simulink model "Collision_avoidance"  (R2020a)
settings: Solver=FixedStepAuto  StartTime=0.0  StopTime=180  FixedStep=0.01  RelTol=1e-3
libraries: simulink x2
settings Model: Creator=Santo  LastModifiedBy=apoor
settings DataIOCC: ReturnWorkspaceOutputs=off
settings OptimizationCC: LifeSpan=inf
settings DebuggingCC: ArithmeticOperatorsInVariantConditions=warning
settings HardwareCC: ProdBitPerSizeT=32  ProdBitPerPtrDiffT=32  ProdWordSize=32  ProdHWDeviceType=Specified
settings SFSimCC: SimUseLocalCustomCode=off  CustomCodeUndefinedFunction=UseInterfaceOnly
settings RTWCC: RTWUseLocalCustomCode=off
settings CodeAppCC: StateflowObjectComments=on

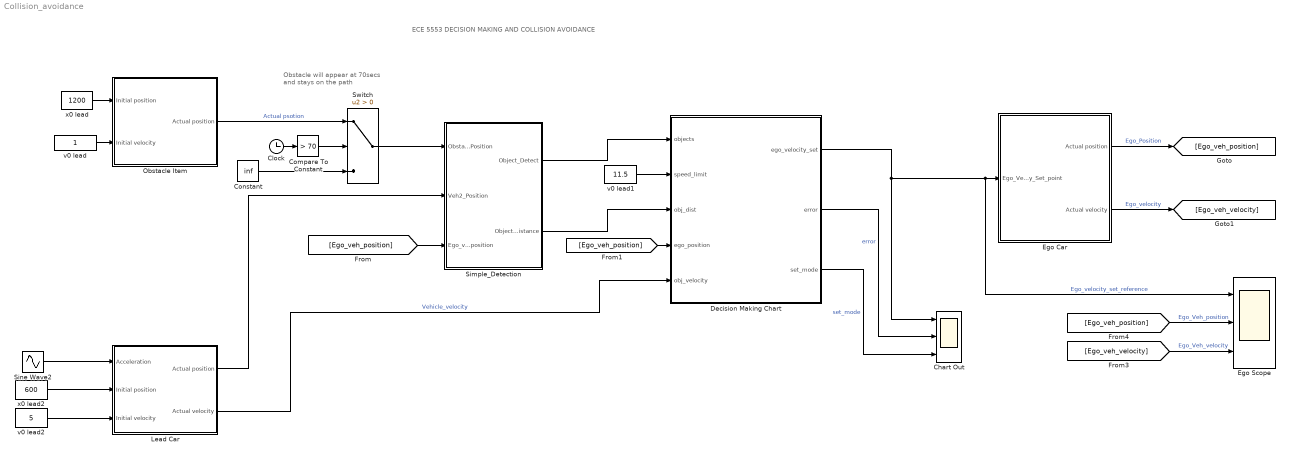
== system Collision_avoidance ==
  note: ECE 5553 DECISION MAKING AND COLLISION AVOIDANCE
  note: Obstacle will appear at 70secs and stays on the path
  Chart Out : Scope  NumInputPorts=3
  Clock : Clock
  Compare To Constant : simulink/Logic and Bit Operations/Compare To Constant  relop=>  const=70  OutDataTypeStr=boolean
  Constant : Constant  Value=inf
  Decision Making Chart : Stateflow chart  TreatAsAtomicUnit=on
  Ego Car : Subsystem
  Ego Scope : Scope  NumInputPorts=3
  Lead Car : Subsystem
  Obstacle Item : Subsystem
  Simple_Detection : Subsystem
  Sine Wave2 : Sin  Amplitude=5  Frequency=0.5  SampleTime=0
  Switch : Switch  Criteria=u2 > Threshold
  v0 lead : Constant  SampleTime=0
  v0 lead1 : Constant  Value=11.5  SampleTime=0
  v0 lead2 : Constant  Value=5  SampleTime=0
  x0 lead : Constant  Value=1200  SampleTime=0
  x0 lead2 : Constant  Value=600  SampleTime=0
  wires:
  x0 lead/1 -> Obstacle Item/1(Initial position)
  v0 lead/1 -> Obstacle Item/2(Initial velocity)
  Lead Car/1(Actual position) -> Simple_Detection/2(Veh2_Position)
  x0 lead2/1 -> Lead Car/2(Initial position)
  v0 lead2/1 -> Lead Car/3(Initial velocity)
  Sine Wave2/1 -> Lead Car/1(Acceleration)
  Simple_Detection/1(Object_Detect) -> Decision Making Chart/1(objects)
  v0 lead1/1 -> Decision Making Chart/2(speed_limit)
  Decision Making Chart/1(ego_velocity_set) -> Chart Out/1, Ego Scope/1, Ego Car/1(Ego_Velocity_Set_point)  "Ego_velocity_set_reference"
  Ego Car/1(Actual position) -> [Ego_veh_position]  "Ego_Position"
  Ego Car/2(Actual velocity) -> [Ego_veh_velocity]  "Ego_velocity"
  Simple_Detection/2(Object_Relative_Distance) -> Decision Making Chart/3(obj_dist)
  Decision Making Chart/2(error) -> Chart Out/2  "error"
  [Ego_veh_position] -> Simple_Detection/3(Ego_veh_position)
  [Ego_veh_position] -> Decision Making Chart/4(ego_position)
  [Ego_veh_velocity] -> Ego Scope/3  "Ego_Veh_velocity"
  [Ego_veh_position] -> Ego Scope/2  "Ego_Veh_position"
  Decision Making Chart/3(set_mode) -> Chart Out/3  "set_mode"
  Lead Car/2(Actual velocity) -> Decision Making Chart/5(obj_velocity)  "Vehicle_velocity"
  Compare To Constant/1 -> Switch/2
  Switch/1 -> Simple_Detection/1(Obstacle_Position)
  Obstacle Item/1(Actual position) -> Switch/1  "Actual psotion"
  Constant/1 -> Switch/3
  Clock/1 -> Compare To Constant/1

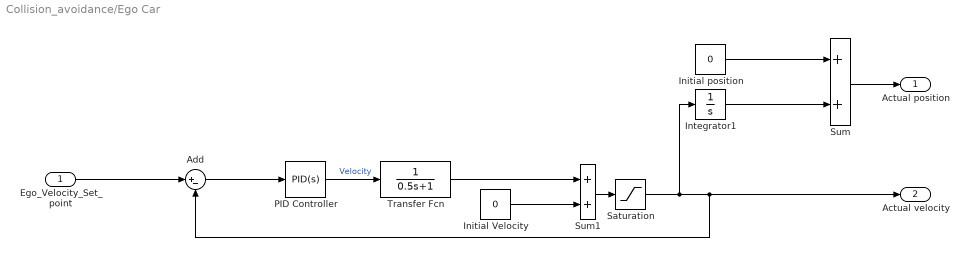
== system Collision_avoidance/Ego Car ==
  Ego_Velocity_Set_point : Inport
  Add : Sum  Inputs=|+-
  Initial Velocity : Constant  Value=0
  Initial position : Constant  Value=0
  Integrator1 : Integrator
  PID Controller : simulink/Continuous/PID Controller  Controller=PID  Form=Parallel  TimeDomain=Continuous-time  UseExternalTs=off  SampleTime=-1  IntegratorMethod=Forward Euler  FilterMethod=Forward Euler  ControllerParametersSource=internal  P=0.543871188851985  I=1.5579001255467  D=0  UseFilter=on  N=100  TunerSelectOption=Transfer Function Based (PID Tuner App)  InitialConditionSource=internal  InitialConditionForIntegrator=0  InitialConditionForFilter=0  DifferentiatorICPrevScaledInput=0  ExternalReset=none  TrackingMode=off  Kt=1  LimitOutput=off  UpperSaturationLimit=inf  LowerSaturationLimit=-inf  LinearizeAsGain=on  AntiWindupMode=none  Kb=1  POutMin=[]  POutMax=[]  IOutMin=[]  IOutMax=[]  DOutMin=[]  DOutMax=[]  NOutMin=[]  NOutMax=[]  SumOutMin=[]  SumOutMax=[]  SaturationOutMin=[]  SaturationOutMax=[]  PParamMin=[]  PParamMax=[]  IParamMin=[]  IParamMax=[]  DParamMin=[]  DParamMax=[]  NParamMin=[]  NParamMax=[]  KbParamMin=[]  KbParamMax=[]  KtParamMin=[]  KtParamMax=[]  KbOutMin=[]  KbOutMax=[]  KtOutMin=[]  KtOutMax=[]  IntegratorOutMin=[]  IntegratorOutMax=[]  FilterOutMin=[]  FilterOutMax=[]  SumI1OutMin=[]  SumI1OutMax=[]  SumI2OutMin=[]  SumI2OutMax=[]  SumI3OutMin=[]  SumI3OutMax=[]  SumI4OutMin=[]  SumI4OutMax=[]  SumDOutMin=[]  SumDOutMax=[]  DifferentiatorOutMin=[]  DifferentiatorOutMax=[]  FilterDiffOutCoefMin=[]  FilterDiffOutCoefMax=[]  ReciprocalOutMin=[]  ReciprocalOutMax=[]  SumDenOutMin=[]  SumDenOutMax=[]  SumNumOutMin=[]  SumNumOutMax=[]  DivideOutMin=[]  DivideOutMax=[]  UdiffTsProdOutMin=[]  UdiffTsProdOutMax=[]  NTsProdOutMin=[]  NTsProdOutMax=[]  UintegralTsProdOutMin=[]  UintegralTsProdOutMax=[]  UngainTsProdOutMin=[]  UngainTsProdOutMax=[]  IntegratorContinuousStateAttributes=''  IntegratorStateMustResolveToSignalObject=off  IntegratorRTWStateStorageClass=Auto  FilterContinuousStateAttributes=''  FilterStateMustResolveToSignalObject=off  FilterRTWStateStorageClass=Auto  ParallelPVariant=InternalParameters  IdealPVariant=Disabled  IVariant=InternalParameters  DVariant=InternalParameters  IntegratorVariant=Continuous  SatVariant=Disabled  AWVariant=Passthrough  PCopyVariant=Disabled  TRVariant=Disabled  FdbkBlocksVariant=Forward  IdealPFdbkVariant=Disabled  SatFdbkVariant=Disabled  DerivativeFilterVariant=ContFilter  NVariant=InternalParameters  NCopyVariant=Disabled  FilterICVariant=InternalICsFilter  IntegratorICVariant=InternalICs  ExternalResetVariant=Disabled  TRSumVariant=Passthrough  SumFdbkVariant=Disabled  SumVariant=Sum_PID  TsampFilterVariant=InternalTs  TsampNgainVariant=Passthrough  TsampIntegralVariant=Passthrough
  Saturation : Saturate  UpperLimit=inf  LowerLimit=0
  Sum : Sum
  Sum1 : Sum
  Transfer Fcn : TransferFcn  Denominator=[0.5 1]
  Actual position : Outport
  Actual velocity : Outport  Port=2
  wires:
  Transfer Fcn/1 -> Sum1/1
  Initial Velocity/1 -> Sum1/2
  Sum/1 -> Actual position/1
  Sum1/1 -> Saturation/1
  PID Controller/1 -> Transfer Fcn/1  "Velocity"
  Initial position/1 -> Sum/1
  Integrator1/1 -> Sum/2
  Add/1 -> PID Controller/1
  Ego_Velocity_Set_point/1 -> Add/1
  Saturation/1 -> Integrator1/1, Add/2, Actual velocity/1

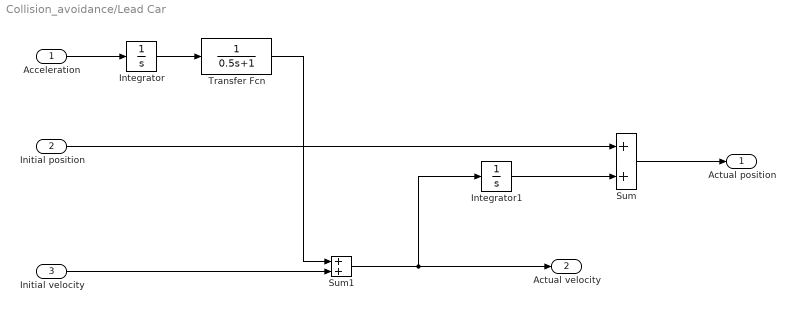
== system Collision_avoidance/Lead Car ==
  Acceleration : Inport
  Initial position : Inport  Port=2
  Initial velocity : Inport  Port=3
  Integrator : Integrator
  Integrator1 : Integrator
  Sum : Sum
  Sum1 : Sum
  Transfer Fcn : TransferFcn  Denominator=[0.5 1]
  Actual position : Outport
  Actual velocity : Outport  Port=2
  wires:
  Integrator1/1 -> Sum/2
  Initial position/1 -> Sum/1
  Acceleration/1 -> Integrator/1
  Sum1/1 -> Actual velocity/1, Integrator1/1
  Integrator/1 -> Transfer Fcn/1
  Sum/1 -> Actual position/1
  Initial velocity/1 -> Sum1/2
  Transfer Fcn/1 -> Sum1/1

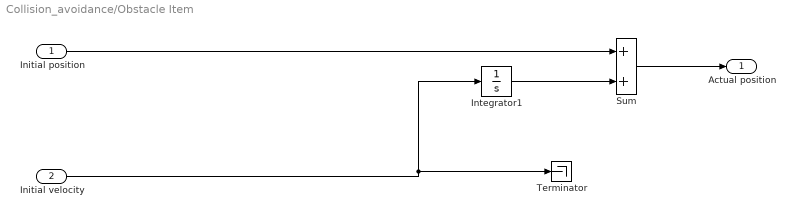
== system Collision_avoidance/Obstacle Item ==
  Initial position : Inport
  Initial velocity : Inport  Port=2
  Integrator1 : Integrator
  Sum : Sum
  Terminator : Terminator
  Actual position : Outport
  wires:
  Sum/1 -> Actual position/1
  Initial velocity/1 -> Terminator/1, Integrator1/1
  Initial position/1 -> Sum/1
  Integrator1/1 -> Sum/2

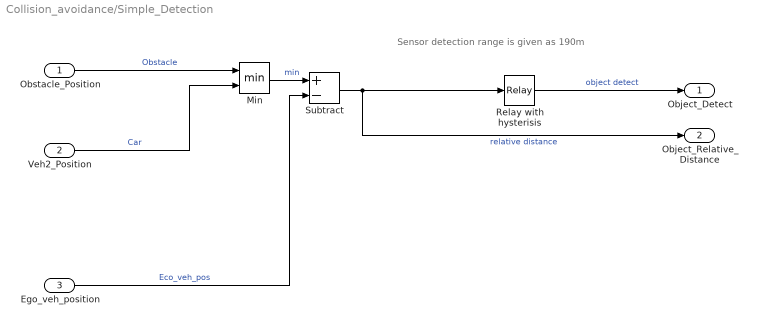
== system Collision_avoidance/Simple_Detection ==
  note: Sensor detection range is given as 190m
  Obstacle_Position : Inport
  Veh2_Position : Inport  Port=2
  Ego_veh_position : Inport  Port=3
  Min : MinMax  Inputs=2
  Relay with hysterisis : Relay  OnSwitchValue=210  OffSwitchValue=190  OnOutputValue=0  OffOutputValue=1
  Subtract : Sum  Inputs=+-
  Object_Detect : Outport
  Object_Relative_Distance : Outport  Port=2
  wires:
  Obstacle_Position/1 -> Min/1  "Obstacle"
  Veh2_Position/1 -> Min/2  "Car"
  Min/1 -> Subtract/1  "min"
  Ego_veh_position/1 -> Subtract/2  "Eco_veh_pos"
  Subtract/1 -> Relay with hysterisis/1, Object_Relative_Distance/1  "relative distance"
  Relay with hysterisis/1 -> Object_Detect/1  "object detect"

== stateflow chart Collision_avoidance/Decision Making Chart ==
  state Follow_Speed_Limit
    ego_velocity_set=speed_limit;
    set_mode=0;
  state objects
  state Lead_Velocity1
    ego_velocity_set=obj_velocity;
    set_mode=1
  state Relative_Distance
    error=obj_dist;
  state LeadCar_Velocity2
    ego_velocity_set=speed_limit;
    set_mode=1;
  state Emergency_stop
    ego_velocity_set=0;
    set_mode=2;
  (default) -> objects
  objects -> Follow_Speed_Limit [order 1] : [objects==0]
  Emergency_stop -> objects
  Follow_Speed_Limit -> objects
  objects -> Relative_Distance [order 2] : [objects==1]
  LeadCar_Velocity2 -> objects
  Lead_Velocity1 -> objects
  Relative_Distance -> (junction 66) [order 2] : [error>50]
  (junction 66) -> Lead_Velocity1 [order 1] : [obj_velocity<speed_limit]
  (junction 66) -> LeadCar_Velocity2 [order 2] : [obj_velocity>speed_limit]
  Relative_Distance -> Emergency_stop [order 1] : [error<=50]
  data: objects input; speed_limit input; ego_velocity_set output; obj_dist input; ego_position input; error output; set_mode output; obj_velocity input
